simulink model "Example3Heart"  (R2025b)
settings: Solver=VariableStepAuto  StartTime=0.0  StopTime=10.0  RelTol=1e-3
libraries: Libs x12
settings Model: Creator=rfen801  LastModifiedBy=rfen801

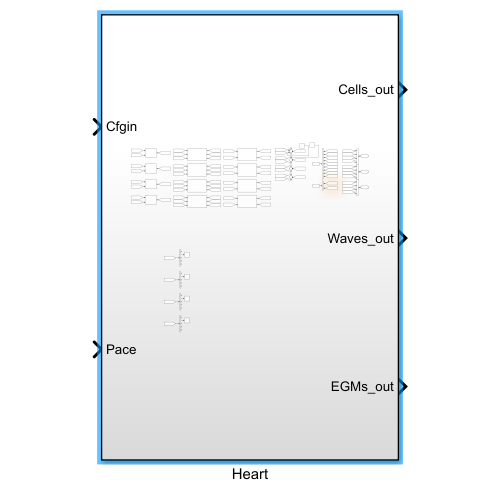
[thumbnail: Simulink's stored preview of the top-level diagram]
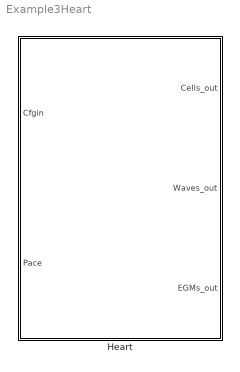
== system Example3Heart ==
  Heart : Subsystem

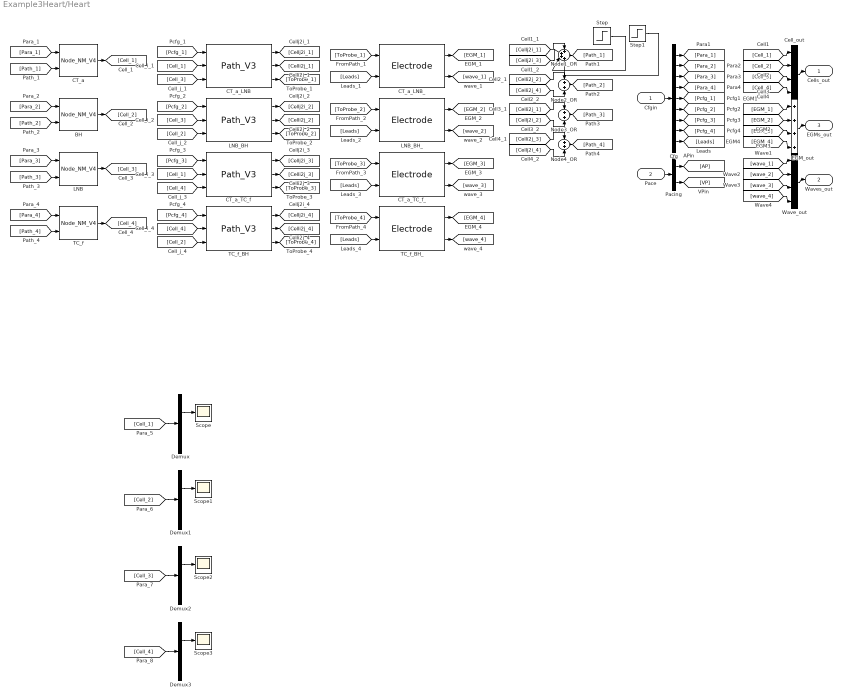
== system Example3Heart/Heart ==
  Cfgin : Inport
  Pace : Inport  Port=2
  BH : Libs/Node_NM_V4  SystemSampleTime=-1  VariantActivationTime=update diagram  EmptyChoice=off  PassThrough=off  PassThroughVariantControl=(default)  EmptyChoiceVariantControl=(default)  AllowFlexibleInterface=on  Latency=0  AutoFrameSizeCalculation=off
  CT_a : Libs/Node_NM_V4  SystemSampleTime=-1  VariantActivationTime=update diagram  EmptyChoice=off  PassThrough=off  PassThroughVariantControl=(default)  EmptyChoiceVariantControl=(default)  AllowFlexibleInterface=on  Latency=0  AutoFrameSizeCalculation=off
  CT_a_LNB : Libs/Path_V3  SystemSampleTime=-1  VariantActivationTime=update diagram  EmptyChoice=off  PassThrough=off  PassThroughVariantControl=(default)  EmptyChoiceVariantControl=(default)  AllowFlexibleInterface=on  Latency=0  AutoFrameSizeCalculation=off
  CT_a_LNB_ : Libs/Electrode  SystemSampleTime=-1  VariantActivationTime=update diagram  EmptyChoice=off  PassThrough=off  PassThroughVariantControl=(default)  EmptyChoiceVariantControl=(default)  AllowFlexibleInterface=on  Latency=0  AutoFrameSizeCalculation=off
  CT_a_TC_f : Libs/Path_V3  SystemSampleTime=-1  VariantActivationTime=update diagram  EmptyChoice=off  PassThrough=off  PassThroughVariantControl=(default)  EmptyChoiceVariantControl=(default)  AllowFlexibleInterface=on  Latency=0  AutoFrameSizeCalculation=off
  CT_a_TC_f_ : Libs/Electrode  SystemSampleTime=-1  VariantActivationTime=update diagram  EmptyChoice=off  PassThrough=off  PassThroughVariantControl=(default)  EmptyChoiceVariantControl=(default)  AllowFlexibleInterface=on  Latency=0  AutoFrameSizeCalculation=off
  Cell_out : Mux
  Cfg : Demux  Outputs=[23,50,50,50,11,11,11,11,28]
  Demux{,1..3} (4 alike) : Demux  Outputs=5
  EGM_out : Sum  Inputs=4
  LNB : Libs/Node_NM_V4  SystemSampleTime=-1  VariantActivationTime=update diagram  EmptyChoice=off  PassThrough=off  PassThroughVariantControl=(default)  EmptyChoiceVariantControl=(default)  AllowFlexibleInterface=on  Latency=0  AutoFrameSizeCalculation=off
  LNB_BH : Libs/Path_V3  SystemSampleTime=-1  VariantActivationTime=update diagram  EmptyChoice=off  PassThrough=off  PassThroughVariantControl=(default)  EmptyChoiceVariantControl=(default)  AllowFlexibleInterface=on  Latency=0  AutoFrameSizeCalculation=off
  LNB_BH_ : Libs/Electrode  SystemSampleTime=-1  VariantActivationTime=update diagram  EmptyChoice=off  PassThrough=off  PassThroughVariantControl=(default)  EmptyChoiceVariantControl=(default)  AllowFlexibleInterface=on  Latency=0  AutoFrameSizeCalculation=off
  Node1_OR : Sum  Inputs=4
  Node2_OR : Sum  Inputs=2
  Node3_OR : Sum  Inputs=2
  Node4_OR : Sum  Inputs=2
  Pacing : Demux  Outputs=2
  Scope{,1..3} (4 alike) : Scope
      Scope settings: ActiveDisplayYMinimum=-14.055953139718371  ActiveDisplayYMaximum=126.50357825746536
      Scope1 settings: ActiveDisplayYMinimum=-16.387499999999996  ActiveDisplayYMaximum=147.48749999999998
      Scope2 settings: ActiveDisplayYMinimum=-16.387499999999996  ActiveDisplayYMaximum=147.48749999999998  DataLoggingVariableName=ScopeData2
      Scope3 settings: ActiveDisplayYMinimum=-14.055953139718371  ActiveDisplayYMaximum=126.50357825746536  DataLoggingVariableName=ScopeData3
  Step : Step  Time=3.32  After=120  SampleTime=0
  Step1 : Step  Time=3.36  After=-120  SampleTime=0
  TC_f : Libs/Node_NM_V4  SystemSampleTime=-1  VariantActivationTime=update diagram  EmptyChoice=off  PassThrough=off  PassThroughVariantControl=(default)  EmptyChoiceVariantControl=(default)  AllowFlexibleInterface=on  Latency=0  AutoFrameSizeCalculation=off
  TC_f_BH : Libs/Path_V3  SystemSampleTime=-1  VariantActivationTime=update diagram  EmptyChoice=off  PassThrough=off  PassThroughVariantControl=(default)  EmptyChoiceVariantControl=(default)  AllowFlexibleInterface=on  Latency=0  AutoFrameSizeCalculation=off
  TC_f_BH_ : Libs/Electrode  SystemSampleTime=-1  VariantActivationTime=update diagram  EmptyChoice=off  PassThrough=off  PassThroughVariantControl=(default)  EmptyChoiceVariantControl=(default)  AllowFlexibleInterface=on  Latency=0  AutoFrameSizeCalculation=off
  Wave_out : Mux
  Cells_out : Outport
  Waves_out : Outport  Port=2
  EGMs_out : Outport  Port=3
  wires:
  CT_a/1 -> [Cell_1]
  [Para_1] -> CT_a/1
  [Path_1] -> CT_a/2
  BH/1 -> [Cell_2]
  [Para_2] -> BH/1
  [Path_2] -> BH/2
  LNB/1 -> [Cell_3]
  [Para_3] -> LNB/1
  [Path_3] -> LNB/2
  TC_f/1 -> [Cell_4]
  [Para_4] -> TC_f/1
  [Path_4] -> TC_f/2
  CT_a_LNB/1 -> [Cellj2i_1]
  CT_a_LNB/2 -> [Celli2j_1]
  CT_a_LNB/3 -> [ToProbe_1]
  [Pcfg_1] -> CT_a_LNB/1
  [Cell_1] -> CT_a_LNB/2
  [Cell_3] -> CT_a_LNB/3
  LNB_BH/1 -> [Cellj2i_2]
  LNB_BH/2 -> [Celli2j_2]
  LNB_BH/3 -> [ToProbe_2]
  [Pcfg_2] -> LNB_BH/1
  [Cell_3] -> LNB_BH/2
  [Cell_2] -> LNB_BH/3
  CT_a_TC_f/1 -> [Cellj2i_3]
  CT_a_TC_f/2 -> [Celli2j_3]
  CT_a_TC_f/3 -> [ToProbe_3]
  [Pcfg_3] -> CT_a_TC_f/1
  [Cell_1] -> CT_a_TC_f/2
  [Cell_4] -> CT_a_TC_f/3
  TC_f_BH/1 -> [Cellj2i_4]
  TC_f_BH/2 -> [Celli2j_4]
  TC_f_BH/3 -> [ToProbe_4]
  [Pcfg_4] -> TC_f_BH/1
  [Cell_4] -> TC_f_BH/2
  [Cell_2] -> TC_f_BH/3
  CT_a_LNB_/1 -> [EGM_1]
  CT_a_LNB_/2 -> [wave_1]
  [ToProbe_1] -> CT_a_LNB_/1
  [Leads] -> CT_a_LNB_/2
  LNB_BH_/1 -> [EGM_2]
  LNB_BH_/2 -> [wave_2]
  [ToProbe_2] -> LNB_BH_/1
  [Leads] -> LNB_BH_/2
  CT_a_TC_f_/1 -> [EGM_3]
  CT_a_TC_f_/2 -> [wave_3]
  [ToProbe_3] -> CT_a_TC_f_/1
  [Leads] -> CT_a_TC_f_/2
  TC_f_BH_/1 -> [EGM_4]
  TC_f_BH_/2 -> [wave_4]
  [ToProbe_4] -> TC_f_BH_/1
  [Leads] -> TC_f_BH_/2
  [Cellj2i_1] -> Node1_OR/1
  [Cellj2i_3] -> Node1_OR/2
  Node1_OR/1 -> [Path_1]
  [Celli2j_2] -> Node2_OR/1
  [Celli2j_4] -> Node2_OR/2
  Node2_OR/1 -> [Path_2]
  [Celli2j_1] -> Node3_OR/1
  [Cellj2i_2] -> Node3_OR/2
  Node3_OR/1 -> [Path_3]
  [Celli2j_3] -> Node4_OR/1
  [Cellj2i_4] -> Node4_OR/2
  Node4_OR/1 -> [Path_4]
  Cfgin/1 -> Cfg/1
  Pace/1 -> Pacing/1
  Cfg/1 -> [Para_1]
  Cfg/2 -> [Para_2]
  Cfg/3 -> [Para_3]
  Cfg/4 -> [Para_4]
  Cfg/5 -> [Pcfg_1]
  Cfg/6 -> [Pcfg_2]
  Cfg/7 -> [Pcfg_3]
  Cfg/8 -> [Pcfg_4]
  Cfg/9 -> [Leads]
  Pacing/1 -> [AP]
  Pacing/2 -> [VP]
  Cell_out/1 -> Cells_out/1
  EGM_out/1 -> EGMs_out/1
  Wave_out/1 -> Waves_out/1
  [Cell_1] -> Cell_out/1
  [Cell_2] -> Cell_out/2
  [Cell_3] -> Cell_out/3
  [Cell_4] -> Cell_out/4
  [EGM_1] -> EGM_out/1
  [EGM_2] -> EGM_out/2
  [EGM_3] -> EGM_out/3
  [EGM_4] -> EGM_out/4
  [wave_1] -> Wave_out/1
  [wave_2] -> Wave_out/2
  [wave_3] -> Wave_out/3
  [wave_4] -> Wave_out/4
  Step/1 -> Node1_OR/3
  Step1/1 -> Node1_OR/4
  Demux2/2 -> Scope2/1
  [Cell_3] -> Demux2/1
  Demux3/2 -> Scope3/1
  [Cell_4] -> Demux3/1
  Demux/2 -> Scope/1
  [Cell_2] -> Demux1/1
  [Cell_1] -> Demux/1
  Demux1/2 -> Scope1/1
